simulink library "Combustion_Calculation"  (R2018b)
settings: Solver=ode45  StartTime=0.0  StopTime=10.0  RelTol=1e-3  EnableMultiTasking=on
settings Model: Creator=drhf  LastModifiedBy=P41573
settings DataIOCC: LimitDataPoints=on  SaveFormat=Array  SignalLoggingSaveFormat=ModelDataLogs
settings OptimizationCC: ExpressionDepthLimit=2147483647  LifeSpan=inf
settings DebuggingCC: UnderspecifiedInitializationDetection=Classic  MergeDetectMultiDrivingBlocksExec=none  SolverPrmCheckMsg=warning  FcnCallInpInsideContextMsg=warning  StateNameClashWarn=warning  SFUnexpectedBacktrackingDiag=warning  SFNoUnconditionalDefaultTransitionDiag=warning  SFExecutionAtInitializationDiag=none
settings HardwareCC: ProdBitPerPointer=32  ProdBitPerSizeT=32  ProdBitPerPtrDiffT=32  ProdLargestAtomicFloat=None  ProdIntDivRoundTo=Undefined  ProdEndianess=Unspecified  ProdWordSize=32  ProdHWDeviceType=32-bit Generic
settings ModelReferenceCC: PropagateSignalLabelsOutOfModel=off
settings SFSimCC: SimUseLocalCustomCode=off
settings RTWCC: RTWUseLocalCustomCode=off
settings CodeAppCC: StateflowObjectComments=on
settings GRTTargetCC: TargetLangStandard=C89/C90 (ANSI)  GeneratePreprocessorConditionals=Disable all  CombineOutputUpdateFcns=off  GRTInterface=on
settings ConfigComp: CovMetricSettings=dw  CovHtmlReporting=on  CovSaveCumulativeToWorkspaceVar=on  CovSaveSingleToWorkspaceVar=on  CovExternalEMLEnable=off

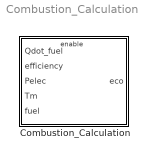
== system Combustion_Calculation ==
  Combustion_Calculation : Subsystem  TreatAsAtomicUnit=on

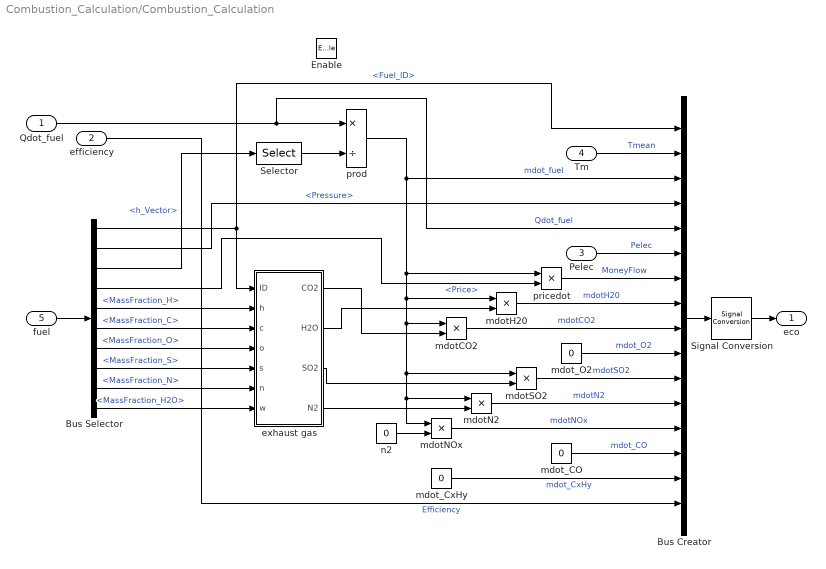
== system Combustion_Calculation/Combustion_Calculation ==
  Qdot_fuel : Inport
  efficiency : Inport  Port=2
  Pelec : Inport  Port=3
  Tm : Inport  Port=4
  fuel : Inport  Port=5
  Enable : EnablePort
  Bus Creator : BusCreator  Inputs=16
  Bus Selector : BusSelector  OutputSignals=Fuel_ID,Pressure,h_Vector,Price,MassFraction_H,MassFraction_C,MassFraction_O,MassFraction_S,MassFraction_N,MassFraction_H2O
  Selector : Selector  IndexOptions=Index vector (dialog)  Indices=[1]  OutputSizes=1
  Signal Conversion : SignalConversion  OverrideOpt=off
  exhaust gas : Subsystem
  mdotCO2 : Product  SaturateOnIntegerOverflow=on  InputSameDT=on  OutDataTypeStr=Inherit: Same as first input
  mdotH20 : Product  SaturateOnIntegerOverflow=on  InputSameDT=on  OutDataTypeStr=Inherit: Same as first input
  mdotN2 : Product  SaturateOnIntegerOverflow=on  InputSameDT=on  OutDataTypeStr=Inherit: Same as first input
  mdotNOx : Product  SaturateOnIntegerOverflow=on  InputSameDT=on  OutDataTypeStr=Inherit: Same as first input
  mdotSO2 : Product  SaturateOnIntegerOverflow=on  InputSameDT=on  OutDataTypeStr=Inherit: Same as first input
  mdot_CO : Constant  Value=0
  mdot_CxHy : Constant  Value=0
  mdot_O2 : Constant  Value=0
  n2 : Constant  Value=0
  pricedot : Product  SaturateOnIntegerOverflow=on  InputSameDT=on  OutDataTypeStr=Inherit: Same as first input
  prod : Product  Inputs=*/  SaturateOnIntegerOverflow=on  InputSameDT=on  OutDataTypeStr=Inherit: Same as first input
  eco : Outport  InitialOutput=0
  wires:
  Signal Conversion/1 -> eco/1
  Selector/1 -> prod/2
  efficiency/1 -> Bus Creator/16  "Efficiency"
  fuel/1 -> Bus Selector/1
  Bus Selector/3 -> Selector/1  "<h_Vector>"
  Bus Creator/1 -> Signal Conversion/1
  Pelec/1 -> Bus Creator/6  "Pelec"
  pricedot/1 -> Bus Creator/7  "MoneyFlow"
  mdotH20/1 -> Bus Creator/8  "mdotH20"
  mdotCO2/1 -> Bus Creator/9  "mdotCO2"
  mdot_O2/1 -> Bus Creator/10  "mdot_O2"
  mdotSO2/1 -> Bus Creator/11  "mdotSO2"
  mdotNOx/1 -> Bus Creator/13  "mdotNOx"
  mdot_CO/1 -> Bus Creator/14  "mdot_CO"
  mdot_CxHy/1 -> Bus Creator/15  "mdot_CxHy"
  Bus Selector/4 -> pricedot/2  "<Price>"
  prod/1 -> pricedot/1, mdotH20/1, mdotCO2/1, mdotSO2/1, mdotNOx/1, mdotN2/1, Bus Creator/3  "mdot_fuel"
  Bus Selector/1 -> exhaust gas/1(ID), Bus Creator/1  "<Fuel_ID>"
  Bus Selector/2 -> Bus Creator/4  "<Pressure>"
  Bus Selector/5 -> exhaust gas/2(h)  "<MassFraction_H>"
  Bus Selector/6 -> exhaust gas/3(c)  "<MassFraction_C>"
  Bus Selector/7 -> exhaust gas/4(o)  "<MassFraction_O>"
  Bus Selector/8 -> exhaust gas/5(s)  "<MassFraction_S>"
  Bus Selector/9 -> exhaust gas/6(n)  "<MassFraction_N>"
  Bus Selector/10 -> exhaust gas/7(w)  "<MassFraction_H2O>"
  exhaust gas/3(SO2) -> mdotSO2/2
  n2/1 -> mdotNOx/2
  exhaust gas/4(N2) -> mdotN2/2
  exhaust gas/1(CO2) -> mdotCO2/2
  exhaust gas/2(H2O) -> mdotH20/2
  mdotN2/1 -> Bus Creator/12  "mdotN2"
  Qdot_fuel/1 -> prod/1, Bus Creator/5  "Qdot_fuel"
  Tm/1 -> Bus Creator/2  "Tmean"

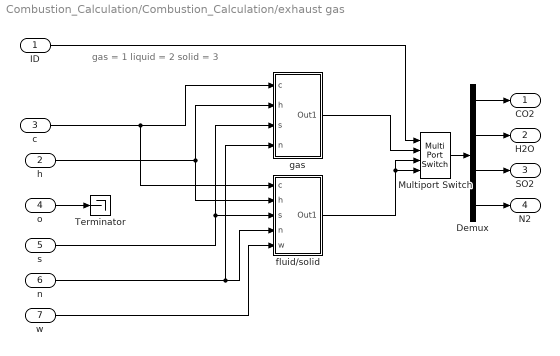
== system Combustion_Calculation/Combustion_Calculation/exhaust gas ==
  note: gas = 1
      | liquid = 2
      | solid = 3
  ID : Inport
  h : Inport  Port=2
  c : Inport  Port=3
  o : Inport  Port=4
  s : Inport  Port=5
  n : Inport  Port=6
  w : Inport  Port=7
  Demux : Demux
  Multiport Switch : MultiPortSwitch  SaturateOnIntegerOverflow=on  InputSameDT=on
  Terminator : Terminator
  fluid/solid : Subsystem
  gas : Subsystem
  CO2 : Outport
  H2O : Outport  Port=2
  SO2 : Outport  Port=3
  N2 : Outport  Port=4
  wires:
  gas/1(Out1) -> Multiport Switch/2
  w/1 -> fluid/solid/5(w)
  o/1 -> Terminator/1
  c/1 -> fluid/solid/1(c), gas/1(c)
  h/1 -> fluid/solid/2(h), gas/2(h)
  n/1 -> fluid/solid/4(n), gas/4(n)
  s/1 -> fluid/solid/3(s), gas/3(s)
  Demux/1 -> CO2/1
  Demux/2 -> H2O/1
  Demux/3 -> SO2/1
  Demux/4 -> N2/1
  Multiport Switch/1 -> Demux/1
  fluid/solid/1(Out1) -> Multiport Switch/3, Multiport Switch/4
  ID/1 -> Multiport Switch/1

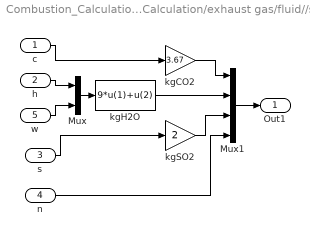
== system Combustion_Calculation/Combustion_Calculation/exhaust gas/fluid//solid ==
  c : Inport
  h : Inport  Port=2
  s : Inport  Port=3
  n : Inport  Port=4
  w : Inport  Port=5
  Mux : Mux  Inputs=2
  Mux1 : Mux
  kgCO2 : Gain  Gain=3.67  SaturateOnIntegerOverflow=on  OutDataTypeStr=Inherit: Same as input  ParamDataTypeStr=Inherit: Same as input
  kgH2O : Fcn  Expr=9*u(1)+u(2)
  kgSO2 : Gain  Gain=2  SaturateOnIntegerOverflow=on  OutDataTypeStr=Inherit: Same as input  ParamDataTypeStr=Inherit: Same as input
  Out1 : Outport
  wires:
  Mux/1 -> kgH2O/1
  kgCO2/1 -> Mux1/1
  kgH2O/1 -> Mux1/2
  kgSO2/1 -> Mux1/3
  c/1 -> kgCO2/1
  h/1 -> Mux/1
  Mux1/1 -> Out1/1
  w/1 -> Mux/2
  s/1 -> kgSO2/1
  n/1 -> Mux1/4

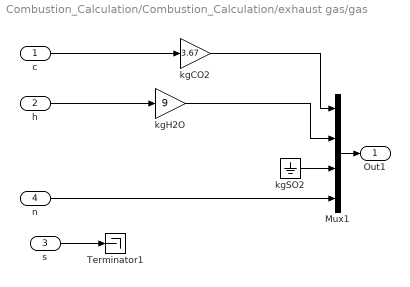
== system Combustion_Calculation/Combustion_Calculation/exhaust gas/gas ==
  c : Inport
  h : Inport  Port=2
  s : Inport  Port=3
  n : Inport  Port=4
  Mux1 : Mux
  Terminator1 : Terminator
  kgCO2 : Gain  Gain=3.67  SaturateOnIntegerOverflow=on  OutDataTypeStr=Inherit: Same as input  ParamDataTypeStr=Inherit: Same as input
  kgH2O : Gain  Gain=9  SaturateOnIntegerOverflow=on  OutDataTypeStr=Inherit: Same as input  ParamDataTypeStr=Inherit: Same as input
  kgSO2 : Ground
  Out1 : Outport
  wires:
  c/1 -> kgCO2/1
  h/1 -> kgH2O/1
  s/1 -> Terminator1/1
  Mux1/1 -> Out1/1
  kgCO2/1 -> Mux1/1
  kgH2O/1 -> Mux1/2
  kgSO2/1 -> Mux1/3
  n/1 -> Mux1/4
